simulink model "version5"  (R2018b)
settings: Solver=FixedStepAuto  StartTime=0.0  StopTime=1  FixedStep=0.0005  RelTol=1e-3  EnableMultiTasking=on
model workspace (MAT data in the model file):
  APPS_1_X = [526 863 1200 1537 1837 2212 2310]
  APPS_2_X = [0 342 684 1026 1368 1710 1805]
  APPS_Y = [100 80 60 40 20 0 0]
  Motor_Temp = [0 25 50 75 85 100 115 125 150 175 200 225 ... (13 elements, 1x13)]
  duty_time = [0 1000 5000 6500 7500 9000 10000 10000 10000 10000 10000 10000 ... (13 elements, 1x13)]
undefined symbols (not defined in the file): I_AN06_5V, I_AN08_5V, I_AN09_5V, I_HALL1, I_SW11_H, O_PWM1_LS0A7, O_PWM2_LS0A7, O_SW01_LS0A4
libraries: ec5744lib x55, simulink x28, canmsglib x12, fuzblock x2
(part 2 of 3)

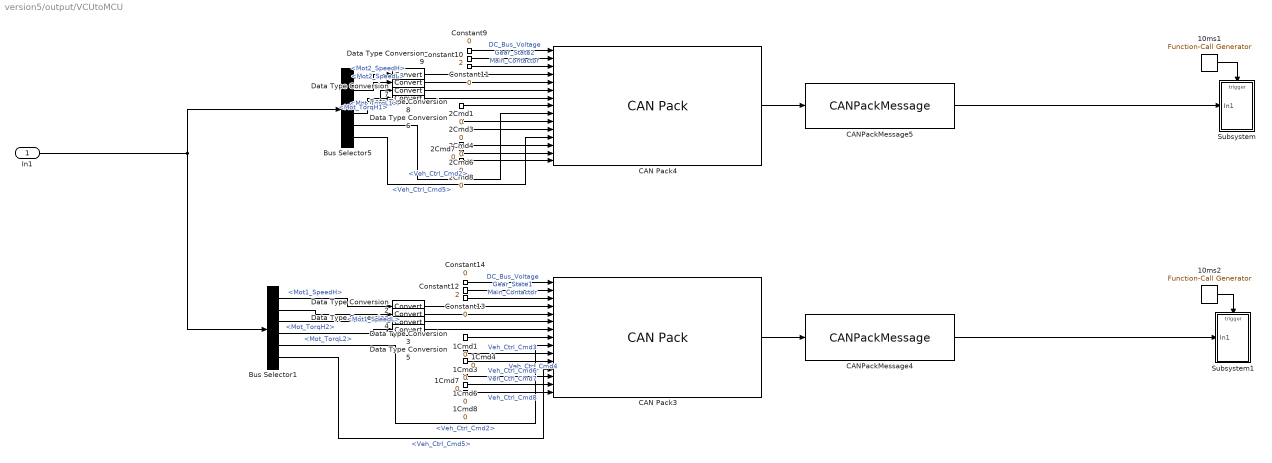
== system version5/output/VCUtoMCU ==
  In1 : Inport
  10ms1 : simulink/Ports & Subsystems/Function-Call Generator  sample_time=0.01  numberOfIterations=1
  10ms2 : simulink/Ports & Subsystems/Function-Call Generator  sample_time=0.01  numberOfIterations=1
  1Cmd{1,3..4,6..8} (6 alike) : Constant  Value=0
  2Cmd{1,3..4,6..8} (6 alike) : Constant  Value=0
  Bus Selector1 : BusSelector  OutputSignals=Mot1_SpeedH,Mot1_SpeedL,Mot_TorqH2,Mot_TorqL2,Veh_Ctrl_Cmd2,Veh_Ctrl_Cmd5
  Bus Selector5 : BusSelector  OutputSignals=Mot2_SpeedH,Mot2_SpeedL,Mot_TorqH1,Mot_TorqL1,Veh_Ctrl_Cmd2,Veh_Ctrl_Cmd5
  CAN Pack3 : canmsglib/CAN Pack  CANdbFile=C:\WH\MC.dbc  MsgList=VCUtoMCU1  MsgName=VCUtoMCU1  MsgIDType=Extended (29-bit identifier)  MsgIdentifier=146927393  MsgLength=8  SignalInfo=DC_Bus_Voltage$48$8$1$2$1$0$1$0$0$255$#Gear_State1$40$2$1$2$1$0$1$0$0$3$#Main_Montactor$43$1$1$2$1$0$1$0$0$1$#Mot1_Sp_H$0$8$1$2$1$0$5.000000e-01$-10000$-10000$-9.872500e+03$#Mot1_Sp_L$8$8$1$2$1$0$1$0$0$255$#Mot1_Torque_H$16$8$1$2$1$0$1$0$0$255$#Mot1_Torque_L$24$8$1$2$1$0$1$0$0$255$#Veh_Ctrl_Cmd1$32$1$1$2$1$0$1$0$0$1$#Veh_Ctrl_Cmd2$33$1$1$2$1$0$1$0$0$1$#Veh_Ctrl_Cmd3$34$1$1$2$1$0$1$0$0$1$#Veh_Ctrl_Cmd4$35$1$1$2$1$0$1$0$0$1$#Veh_Ctrl_Cmd5$36$1$1$2$1$0$1$0$0$1$#Veh_Ctrl_Cmd6$37$1$1$2$1$0$1$0$0$1$#Veh_Ctrl_Cmd7$38$1$1$2$1$0$1$0$0$1$#Veh_Ctrl_Cmd8$39$1$1$2$1$0$1$0$0$1$#  NSignals=15  StartBits=str2num('[int32(48);int32(40);int32(43);int32(0);int32(8);int32(16);int32(24);int32(32);int32(33);int32(34);int32(35);int32(36);int32(37);int32(38);int32(39)]')  SignalSizes=str2num('[int32(8);int32(2);int32(1);int32(8);int32(8);int32(8);int32(8);int32(1);int32(1);int32(1);int32(1);int32(1);int32(1);int32(1);int32(1)]')  ByteOrders=str2num('[int32(1);int32(1);int32(1);int32(1);int32(1);int32(1);int32(1);int32(1);int32(1);int32(1);int32(1);int32(1);int32(1);int32(1);int32(1)]')  DataTypes=str2num('[int32(2);int32(2);int32(2);int32(2);int32(2);int32(2);int32(2);int32(2);int32(2);int32(2);int32(2);int32(2);int32(2);int32(2);int32(2)]')  MultiplexTypes=str2num('[int32(1);int32(1);int32(1);int32(1);int32(1);int32(1);int32(1);int32(1);int32(1);int32(1);int32(1);int32(1);int32(1);int32(1);int32(1)]')  MultiplexValues=str2num('[double(0);double(0);double(0);double(0);double(0);double(0);double(0);double(0);double(0);double(0);double(0);double(0);double(0);double(0);double(0)]')  Factors=str2num('[double(1);double(1);double(1);double(5.000000e-01);double(1);double(1);double(1);double(1);double(1);double(1);double(1);double(1);double(1);double(1);double(1)]')  Offsets=str2num('[double(0);double(0);double(0);double(-10000);double(0);double(0);double(0);double(0);double(0);double(0);double(0);double(0);double(0);double(0);double(0)]')  Minimums=str2num('[double(0);double(0);double(0);double(-10000);double(0);double(0);double(0);double(0);double(0);double(0);double(0);double(0);double(0);double(0);double(0)]')  Maximums=str2num('[double(255);double(3);double(1);double(-9.872500e+03);double(255);double(255);double(255);double(1);double(1);double(1);double(1);double(1);double(1);double(1);double(1)]')  Remote=off  ApplyMinMax=off  BusOutput=off
      settings: SourceProductName=Simulink Real-Time  SourceProductBaseCode=XP  DataFormat=CANdb specified signals
  CAN Pack4 : canmsglib/CAN Pack  CANdbFile=C:\WH\MC.dbc  MsgList=VCUtoMCU2  MsgName=VCUtoMCU2  MsgIDType=Extended (29-bit identifier)  MsgIdentifier=145878817  MsgLength=8  SignalInfo=DC_Bus_Voltage$48$8$1$2$1$0$1$0$0$255$#Gear_State_2$40$2$1$2$1$0$1$0$0$3$#Main_Montactor$43$1$1$2$1$0$1$0$0$1$#Mot2_Sp_H$16$8$1$2$1$0$5.000000e-01$-10000$-10000$-9.872500e+03$#Mot2_Sp_L$24$8$1$2$1$0$5.000000e-01$-10000$-10000$-9.872500e+03$#Mot2_Torque_H$0$8$1$2$1$0$1$0$0$255$#Mot2_Torque_L$8$8$1$2$1$0$1$0$0$255$#Veh_Ctrl_Cmd1$32$1$1$2$1$0$1$0$0$1$#Veh_Ctrl_Cmd2$33$1$1$2$1$0$1$0$0$1$#Veh_Ctrl_Cmd3$34$1$1$2$1$0$1$0$0$1$#Veh_Ctrl_Cmd4$35$1$1$2$1$0$1$0$0$1$#Veh_Ctrl_Cmd5$36$1$1$2$1$0$1$0$0$1$#Veh_Ctrl_Cmd6$37$1$1$2$1$0$1$0$0$1$#Veh_Ctrl_Cmd7$38$1$1$2$1$0$1$0$0$1$#Veh_Ctrl_Cmd8$39$1$1$2$1$0$1$0$0$1$#  NSignals=15  StartBits=str2num('[int32(48);int32(40);int32(43);int32(16);int32(24);int32(0);int32(8);int32(32);int32(33);int32(34);int32(35);int32(36);int32(37);int32(38);int32(39)]')  SignalSizes=str2num('[int32(8);int32(2);int32(1);int32(8);int32(8);int32(8);int32(8);int32(1);int32(1);int32(1);int32(1);int32(1);int32(1);int32(1);int32(1)]')  ByteOrders=str2num('[int32(1);int32(1);int32(1);int32(1);int32(1);int32(1);int32(1);int32(1);int32(1);int32(1);int32(1);int32(1);int32(1);int32(1);int32(1)]')  DataTypes=str2num('[int32(2);int32(2);int32(2);int32(2);int32(2);int32(2);int32(2);int32(2);int32(2);int32(2);int32(2);int32(2);int32(2);int32(2);int32(2)]')  MultiplexTypes=str2num('[int32(1);int32(1);int32(1);int32(1);int32(1);int32(1);int32(1);int32(1);int32(1);int32(1);int32(1);int32(1);int32(1);int32(1);int32(1)]')  MultiplexValues=str2num('[double(0);double(0);double(0);double(0);double(0);double(0);double(0);double(0);double(0);double(0);double(0);double(0);double(0);double(0);double(0)]')  Factors=str2num('[double(1);double(1);double(1);double(5.000000e-01);double(5.000000e-01);double(1);double(1);double(1);double(1);double(1);double(1);double(1);double(1);double(1);double(1)]')  Offsets=str2num('[double(0);double(0);double(0);double(-10000);double(-10000);double(0);double(0);double(0);double(0);double(0);double(0);double(0);double(0);double(0);double(0)]')  Minimums=str2num('[double(0);double(0);double(0);double(-10000);double(-10000);double(0);double(0);double(0);double(0);double(0);double(0);double(0);double(0);double(0);double(0)]')  Maximums=str2num('[double(255);double(3);double(1);double(-9.872500e+03);double(-9.872500e+03);double(255);double(255);double(1);double(1);double(1);double(1);double(1);double(1);double(1);double(1)]')  Remote=off  ApplyMinMax=off  BusOutput=off
      settings: SourceProductName=Simulink Real-Time  SourceProductBaseCode=XP  DataFormat=CANdb specified signals
  CANPackMessage4 : ec5744lib/RapidECU_U3/04CANCommunication/CANPackMessage  datalength=8  sampletime=-1
      settings: SourceProductName=ECUCoder for MPC5744
  CANPackMessage5 : ec5744lib/RapidECU_U3/04CANCommunication/CANPackMessage  datalength=8  sampletime=-1
      settings: SourceProductName=ECUCoder for MPC5744
  Constant10 : Constant  Value=2
  Constant11 : Constant  Value=0
  Constant12 : Constant  Value=2  LockScale=on
  Constant13 : Constant  Value=0
  Constant14 : Constant  Value=0
  Constant9 : Constant  Value=0  OutDataTypeStr=uint8
  Data Type Conversion{2..9} (8 alike) : DataTypeConversion
  Subsystem : Subsystem
  Subsystem1 : Subsystem
  wires:
  Constant13/1 -> CAN Pack3/3  "Main_Contactor"
  1Cmd7/1 -> CAN Pack3/14  "Veh_Ctrl_Cmd7"
  CAN Pack3/1 -> CANPackMessage4/1
  Data Type Conversion2/1 -> CAN Pack3/4
  CAN Pack4/1 -> CANPackMessage5/1
  2Cmd7/1 -> CAN Pack4/14
  Constant10/1 -> CAN Pack4/2  "Gear_State2"
  1Cmd8/1 -> CAN Pack3/15  "Veh_Ctrl_Cmd8"
  2Cmd8/1 -> CAN Pack4/15
  Data Type Conversion5/1 -> CAN Pack3/7
  Constant12/1 -> CAN Pack3/2  "Gear_State1"
  CANPackMessage5/1 -> Subsystem/1(In1)
  2Cmd6/1 -> CAN Pack4/13
  1Cmd4/1 -> CAN Pack3/11  "Veh_Ctrl_Cmd4"
  Data Type Conversion7/1 -> CAN Pack4/6
  Constant14/1 -> CAN Pack3/1  "DC_Bus_Voltage"
  Data Type Conversion3/1 -> CAN Pack3/5
  1Cmd3/1 -> CAN Pack3/10  "Veh_Ctrl_Cmd3"
  Constant9/1 -> CAN Pack4/1  "DC_Bus_Voltage"
  Bus Selector5/5 -> CAN Pack4/9  "<Veh_Ctrl_Cmd2>"
  1Cmd6/1 -> CAN Pack3/13  "Veh_Ctrl_Cmd6"
  10ms2/1 -> Subsystem1/Trigger
  Constant11/1 -> CAN Pack4/3  "Main_Contactor"
  2Cmd4/1 -> CAN Pack4/11
  Bus Selector5/6 -> CAN Pack4/12  "<Veh_Ctrl_Cmd5>"
  In1/1 -> Bus Selector5/1, Bus Selector1/1
  2Cmd1/1 -> CAN Pack4/8
  Bus Selector5/1 -> Data Type Conversion9/1  "<Mot2_SpeedH>"
  CANPackMessage4/1 -> Subsystem1/1(In1)
  Bus Selector1/5 -> CAN Pack3/9  "<Veh_Ctrl_Cmd2>"
  2Cmd3/1 -> CAN Pack4/10
  Data Type Conversion4/1 -> CAN Pack3/6
  10ms1/1 -> Subsystem/Trigger
  Data Type Conversion8/1 -> CAN Pack4/5
  Bus Selector1/3 -> Data Type Conversion4/1  "<Mot_TorqH2>"
  Bus Selector1/4 -> Data Type Conversion5/1  "<Mot_TorqL2>"
  Bus Selector5/4 -> Data Type Conversion6/1  "<Mot_TorqL1>"
  Data Type Conversion9/1 -> CAN Pack4/4
  1Cmd1/1 -> CAN Pack3/8
  Bus Selector1/1 -> Data Type Conversion2/1  "<Mot1_SpeedH>"
  Bus Selector1/2 -> Data Type Conversion3/1  "<Mot1_SpeedL>"
  Bus Selector1/6 -> CAN Pack3/12  "<Veh_Ctrl_Cmd5>"
  Bus Selector5/2 -> Data Type Conversion8/1  "<Mot2_SpeedL>"
  Data Type Conversion6/1 -> CAN Pack4/7
  Bus Selector5/3 -> Data Type Conversion7/1  "<Mot_TorqH1>"

== system version5/control/APS_Ctrl/clock ==
  In1 : Inport
  AND : Logic  IconShape=distinctive  AllPortsSameDT=off  OutDataTypeStr=boolean
  Compare To Constant : simulink/Logic and Bit Operations/Compare To Constant  relop===  const=1  OutDataTypeStr=boolean
  Compare To Constant1 : simulink/Logic and Bit Operations/Compare To Constant  relop===  const=1  OutDataTypeStr=boolean
  计时计数 : Subsystem  Description=计数模块，当有输入信号有跳变的时候会触发使计数值清零  TreatAsAtomicUnit=on
  Out1 : Outport
  wires:
  Compare To Constant1/1 -> AND/2
  Compare To Constant/1 -> AND/1
  计时计数/1(Count_state) -> Compare To Constant/1
  In1/1 -> 计时计数/1(计数状态), Compare To Constant1/1
  AND/1 -> Out1/1

== system version5/control/tcs/0-75直线加速 ==
  In1 : Inport
  In2 : Inport  Port=2
  In3 : Inport  Port=3
  1-D Lookup Table : Lookup_n-D  NumberOfTableDimensions=1  BreakpointsForDimension1=[1 256 512 768 1024 1280 1536 1792 2048 2304 2560 2816 3072 3328 3584 3840 4096 4352 4608 4864 5120 5376 5632 5888 6000]  Table=[134 134 134 134 134 134 134 134 134 134 134 134 134 134 134 134 134 134 132 130 128 125 120 117 115]  InternalRulePriority=Speed  RndMeth=Simplest  InputSameDT=on
  1-D Lookup Table1 : Lookup_n-D  NumberOfTableDimensions=1  BreakpointsForDimension1=[1 256 512 768 1024 1280 1536 1792 2048 2304 2560 2816 3072 3328 3584 3840 4096 4352 4608 4864 5120 5376 5632 5888 6000]  Table=[134 134 134 134 134 134 134 134 134 134 134 134 134 134 134 134 134 134 132 130 128 125 120 117 115]  InternalRulePriority=Speed  RndMeth=Simplest  InputSameDT=on
  "ACC " : Fcn  Expr=u(1)^(0.7)
  Dot Product4 : DotProduct  InputSameDT=on  OutDataTypeStr=Inherit: Inherit via internal rule
  Gain2 : Gain  Gain=0.5  OutDataTypeStr=double
  Subtract1 : Sum  AccumDataTypeStr=double  OutDataTypeStr=uint16  SaturateOnIntegerOverflow=on
  Out1 : Outport
  Output : Outport  Port=2
  wires:
  Dot Product4/1 -> Out1/1
  In2/1 -> 1-D Lookup Table/1
  Subtract1/1 -> Gain2/1
  1-D Lookup Table1/1 -> Subtract1/2
  In3/1 -> 1-D Lookup Table1/1
  "ACC "/1 -> Dot Product4/2
  In1/1 -> "ACC "/1
  1-D Lookup Table/1 -> Subtract1/1
  Gain2/1 -> Output/1, Dot Product4/1

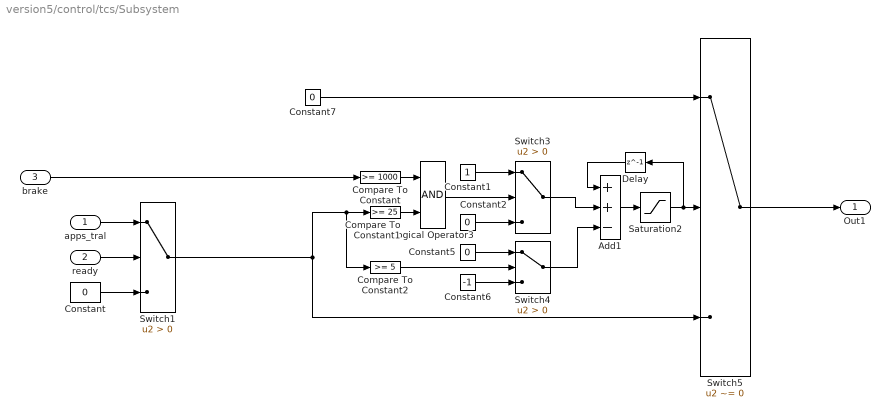
== system version5/control/tcs/Subsystem ==
  apps_tral : Inport
  ready : Inport  Port=2
  brake : Inport  Port=3
  Add1 : Sum  Inputs=++-
  Compare To Constant : simulink/Logic and Bit Operations/Compare To Constant  relop=>=  const=1000  OutDataTypeStr=boolean
  Compare To Constant1 : simulink/Logic and Bit Operations/Compare To Constant  relop=>=  const=25  OutDataTypeStr=boolean
  Compare To Constant2 : simulink/Logic and Bit Operations/Compare To Constant  relop=>=  const=5  OutDataTypeStr=boolean
  Constant{,2,5,7} (4 alike) : Constant  Value=0
  Constant1 : Constant
  Constant6 : Constant  Value=-1
  Delay : Delay  DelayLength=1  InitialCondition=0
  Logical Operator3 : Logic  AllPortsSameDT=off  OutDataTypeStr=boolean
  Saturation2 : Saturate  UpperLimit=1  LowerLimit=0  OutDataTypeStr=single
  Switch1 : Switch  Criteria=u2 > Threshold
  Switch3 : Switch  Criteria=u2 > Threshold  OutDataTypeStr=single
  Switch4 : Switch  Criteria=u2 > Threshold  OutDataTypeStr=single
  Switch5 : Switch  Criteria=u2 ~= 0  OutDataTypeStr=uint16
  Out1 : Outport
  wires:
  Switch4/1 -> Add1/3
  Constant/1 -> Switch1/3
  Switch1/1 -> Compare To Constant2/1, Compare To Constant1/1, Switch5/3
  Constant5/1 -> Switch4/1
  Constant2/1 -> Switch3/3
  apps_tral/1 -> Switch1/1
  Constant6/1 -> Switch4/3
  Delay/1 -> Add1/1
  Compare To Constant1/1 -> Logical Operator3/2
  Add1/1 -> Saturation2/1
  Compare To Constant2/1 -> Switch4/2
  Switch3/1 -> Add1/2
  Compare To Constant/1 -> Logical Operator3/1
  Constant7/1 -> Switch5/1
  Saturation2/1 -> Delay/1, Switch5/2
  Logical Operator3/1 -> Switch3/2
  Constant1/1 -> Switch3/1
  brake/1 -> Compare To Constant/1
  Switch5/1 -> Out1/1
  ready/1 -> Switch1/2

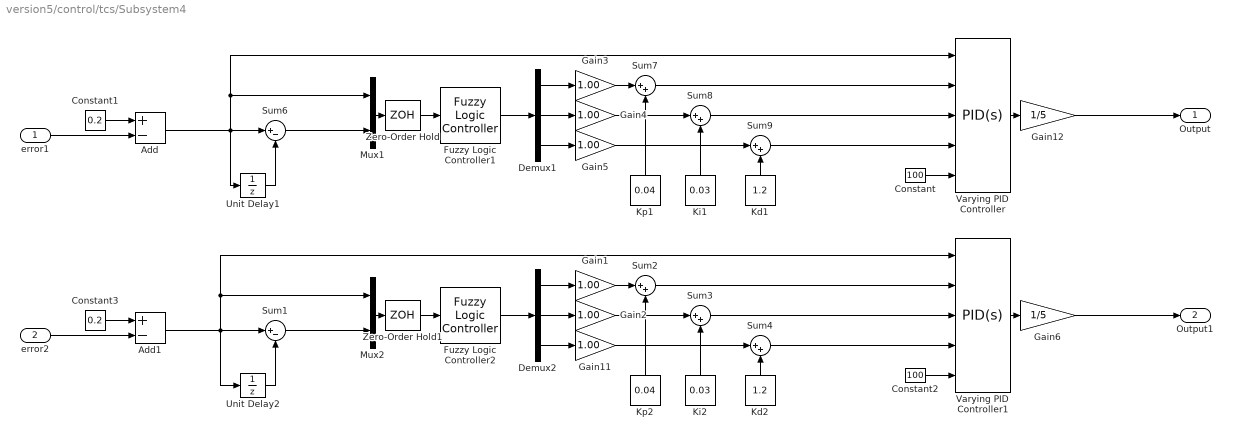
== system version5/control/tcs/Subsystem4 ==
  error1 : Inport
  error2 : Inport  Port=2
  Add : Sum  Inputs=+-
  Add1 : Sum  Inputs=+-
  Constant : Constant  Value=100
  Constant1 : Constant  Value=0.2
  Constant2 : Constant  Value=100
  Constant3 : Constant  Value=0.2
  Demux1 : Demux  Outputs=3
  Demux2 : Demux  Outputs=3
  Fuzzy Logic Controller1 : fuzblock/Fuzzy Logic  Controller  FIS='myfuzzyrules.fis'  OutputSampleNumber=101  DataType=double  FuzzifiedInputs=off  RuleFiringStrengths=off  RuleOutputs=off  AggregatedOutputs=off  SimulateUsing=Interpreted execution  OutOfRangeInputValueMessage=warning  NoRuleFiredMessage=warning  EmptyOutputFuzzySetMessage=warning
  Fuzzy Logic Controller2 : fuzblock/Fuzzy Logic  Controller  FIS='myfuzzyrules.fis'  OutputSampleNumber=101  DataType=double  FuzzifiedInputs=off  RuleFiringStrengths=off  RuleOutputs=off  AggregatedOutputs=off  SimulateUsing=Interpreted execution  OutOfRangeInputValueMessage=warning  NoRuleFiredMessage=warning  EmptyOutputFuzzySetMessage=warning
  Gain{1..5,11} (6 alike) : Gain  Gain=1.00
  Gain12 : Gain  Gain=1/5
  Gain6 : Gain  Gain=1/5
  Kd1 : Constant  Value=1.2
  Kd2 : Constant  Value=1.2
  Ki1 : Constant  Value=0.03
  Ki2 : Constant  Value=0.03
  Kp1 : Constant  Value=0.04
  Kp2 : Constant  Value=0.04
  Mux1 : Mux  Inputs=2
  Mux2 : Mux  Inputs=2
  Sum1 : Sum  Inputs=|+-
  Sum{2..4,7..9} (6 alike) : Sum  Inputs=|++
  Sum6 : Sum  Inputs=|+-
  Unit Delay1 : UnitDelay  SampleTime=-1
  Unit Delay2 : UnitDelay  SampleTime=-1
  Varying PID Controller : simulink/Continuous/PID Controller  Controller=PID  Form=Parallel  TimeDomain=Continuous-time  SampleTime=-1  IntegratorMethod=Forward Euler  FilterMethod=Forward Euler  ControllerParametersSource=external  P=1  I=1  D=0  UseFilter=on  N=100  TunerSelectOption=Transfer Function Based (PID Tuner App)  InitialConditionSource=internal  InitialConditionForIntegrator=0  InitialConditionForFilter=0  DifferentiatorICPrevScaledInput=0  ExternalReset=none  TrackingMode=off  Kt=1  LimitOutput=off  UpperSaturationLimit=inf  LowerSaturationLimit=-inf  LinearizeAsGain=on  AntiWindupMode=none  Kb=1  POutMin=[]  POutMax=[]  IOutMin=[]  IOutMax=[]  DOutMin=[]  DOutMax=[]  NOutMin=[]  NOutMax=[]  SumOutMin=[]  SumOutMax=[]  SaturationOutMin=[]  SaturationOutMax=[]  PParamMin=[]  PParamMax=[]  IParamMin=[]  IParamMax=[]  DParamMin=[]  DParamMax=[]  NParamMin=[]  NParamMax=[]  KbParamMin=[]  KbParamMax=[]  KtParamMin=[]  KtParamMax=[]  KbOutMin=[]  KbOutMax=[]  KtOutMin=[]  KtOutMax=[]  IntegratorOutMin=[]  IntegratorOutMax=[]  FilterOutMin=[]  FilterOutMax=[]  SumI1OutMin=[]  SumI1OutMax=[]  SumI2OutMin=[]  SumI2OutMax=[]  SumI3OutMin=[]  SumI3OutMax=[]  SumI4OutMin=[]  SumI4OutMax=[]  SumDOutMin=[]  SumDOutMax=[]  DifferentiatorOutMin=[]  DifferentiatorOutMax=[]  FilterDiffOutCoefMin=[]  FilterDiffOutCoefMax=[]  ReciprocalOutMin=[]  ReciprocalOutMax=[]  SumDenOutMin=[]  SumDenOutMax=[]  SumNumOutMin=[]  SumNumOutMax=[]  DivideOutMin=[]  DivideOutMax=[]  IntegratorContinuousStateAttributes=''  IntegratorStateMustResolveToSignalObject=off  IntegratorRTWStateStorageClass=Auto  FilterContinuousStateAttributes=''  FilterStateMustResolveToSignalObject=off  FilterRTWStateStorageClass=Auto  ParallelPVariant=ExternalParameters  IdealPVariant=Disabled  IVariant=ExternalParameters  DVariant=ExternalParameters  IntegratorVariant=Continuous  SatVariant=Disabled  AWVariant=Passthrough  PCopyVariant=Disabled  TRVariant=Disabled  FdbkBlocksVariant=Forward  IdealPFdbkVariant=Disabled  SatFdbkVariant=Disabled  DerivativeFilterVariant=ContFilter  NVariant=ExternalParameters  NCopyVariant=Disabled  FilterICVariant=InternalICsFilter  IntegratorICVariant=InternalICs  ExternalResetVariant=Disabled  TRSumVariant=Passthrough  SumFdbkVariant=Disabled  SumVariant=Sum_PID
  Varying PID Controller1 : simulink/Continuous/PID Controller  Controller=PID  Form=Parallel  TimeDomain=Continuous-time  SampleTime=-1  IntegratorMethod=Forward Euler  FilterMethod=Forward Euler  ControllerParametersSource=external  P=1  I=1  D=0  UseFilter=on  N=100  TunerSelectOption=Transfer Function Based (PID Tuner App)  InitialConditionSource=internal  InitialConditionForIntegrator=0  InitialConditionForFilter=0  DifferentiatorICPrevScaledInput=0  ExternalReset=none  TrackingMode=off  Kt=1  LimitOutput=off  UpperSaturationLimit=inf  LowerSaturationLimit=-inf  LinearizeAsGain=on  AntiWindupMode=none  Kb=1  POutMin=[]  POutMax=[]  IOutMin=[]  IOutMax=[]  DOutMin=[]  DOutMax=[]  NOutMin=[]  NOutMax=[]  SumOutMin=[]  SumOutMax=[]  SaturationOutMin=[]  SaturationOutMax=[]  PParamMin=[]  PParamMax=[]  IParamMin=[]  IParamMax=[]  DParamMin=[]  DParamMax=[]  NParamMin=[]  NParamMax=[]  KbParamMin=[]  KbParamMax=[]  KtParamMin=[]  KtParamMax=[]  KbOutMin=[]  KbOutMax=[]  KtOutMin=[]  KtOutMax=[]  IntegratorOutMin=[]  IntegratorOutMax=[]  FilterOutMin=[]  FilterOutMax=[]  SumI1OutMin=[]  SumI1OutMax=[]  SumI2OutMin=[]  SumI2OutMax=[]  SumI3OutMin=[]  SumI3OutMax=[]  SumI4OutMin=[]  SumI4OutMax=[]  SumDOutMin=[]  SumDOutMax=[]  DifferentiatorOutMin=[]  DifferentiatorOutMax=[]  FilterDiffOutCoefMin=[]  FilterDiffOutCoefMax=[]  ReciprocalOutMin=[]  ReciprocalOutMax=[]  SumDenOutMin=[]  SumDenOutMax=[]  SumNumOutMin=[]  SumNumOutMax=[]  DivideOutMin=[]  DivideOutMax=[]  IntegratorContinuousStateAttributes=''  IntegratorStateMustResolveToSignalObject=off  IntegratorRTWStateStorageClass=Auto  FilterContinuousStateAttributes=''  FilterStateMustResolveToSignalObject=off  FilterRTWStateStorageClass=Auto  ParallelPVariant=ExternalParameters  IdealPVariant=Disabled  IVariant=ExternalParameters  DVariant=ExternalParameters  IntegratorVariant=Continuous  SatVariant=Disabled  AWVariant=Passthrough  PCopyVariant=Disabled  TRVariant=Disabled  FdbkBlocksVariant=Forward  IdealPFdbkVariant=Disabled  SatFdbkVariant=Disabled  DerivativeFilterVariant=ContFilter  NVariant=ExternalParameters  NCopyVariant=Disabled  FilterICVariant=InternalICsFilter  IntegratorICVariant=InternalICs  ExternalResetVariant=Disabled  TRSumVariant=Passthrough  SumFdbkVariant=Disabled  SumVariant=Sum_PID
  Zero-Order Hold : ZeroOrderHold  SampleTime=-1
  Zero-Order Hold1 : ZeroOrderHold  SampleTime=-1
  Output : Outport
  Output1 : Outport  Port=2
  wires:
  Sum9/1 -> Varying PID Controller/4
  Gain4/1 -> Sum8/1
  Sum8/1 -> Varying PID Controller/3
  Constant1/1 -> Add/1
  Gain3/1 -> Sum7/1
  Fuzzy Logic Controller1/1 -> Demux1/1
  Demux1/1 -> Gain3/1
  Unit Delay1/1 -> Sum6/2
  Kd1/1 -> Sum9/2
  Demux1/2 -> Gain4/1
  Kp1/1 -> Sum7/2
  Sum7/1 -> Varying PID Controller/2
  Gain5/1 -> Sum9/1
  error1/1 -> Add/2
  Demux1/3 -> Gain5/1
  Ki1/1 -> Sum8/2
  Constant/1 -> Varying PID Controller/5
  Sum2/1 -> Varying PID Controller1/2
  Sum3/1 -> Varying PID Controller1/3
  Sum4/1 -> Varying PID Controller1/4
  Constant3/1 -> Add1/1
  Demux2/2 -> Gain2/1
  Demux2/3 -> Gain11/1
  Unit Delay2/1 -> Sum1/2
  Gain11/1 -> Sum4/1
  Kp2/1 -> Sum2/2
  Demux2/1 -> Gain1/1
  Gain1/1 -> Sum2/1
  Fuzzy Logic Controller2/1 -> Demux2/1
  Ki2/1 -> Sum3/2
  Kd2/1 -> Sum4/2
  Constant2/1 -> Varying PID Controller1/5
  Gain2/1 -> Sum3/1
  Varying PID Controller1/1 -> Gain6/1
  error2/1 -> Add1/2
  Varying PID Controller/1 -> Gain12/1
  Gain12/1 -> Output/1
  Gain6/1 -> Output1/1
  Sum6/1 -> Mux1/2
  Sum1/1 -> Mux2/2
  Add/1 -> Varying PID Controller/1, Mux1/1, Unit Delay1/1, Sum6/1
  Add1/1 -> Mux2/1, Varying PID Controller1/1, Unit Delay2/1, Sum1/1
  Zero-Order Hold/1 -> Fuzzy Logic Controller1/1
  Mux1/1 -> Zero-Order Hold/1
  Zero-Order Hold1/1 -> Fuzzy Logic Controller2/1
  Mux2/1 -> Zero-Order Hold1/1

== system version5/control/tcs/均值滤波器 ==
  In1 : Inport
  Add2 : Sum  Inputs=-+-
  Constant2 : Constant  Value=4  OutDataTypeStr=uint8  SampleTime=-1
  Divide : Product  Inputs=*/
  MinMax : MinMax
  MinMax1 : MinMax  Function=max
  Sum of Elements : Sum  Inputs=+
  Tapped Delay : simulink/Discrete/Tapped Delay  vinit=0.0  samptime=-1  NumDelays=4  DelayOrder=Oldest  includeCurrent=off
  Out1 : Outport
  wires:
  In1/1 -> Tapped Delay/1
  Add2/1 -> Divide/1
  MinMax/1 -> Add2/3
  MinMax1/1 -> Add2/1
  Divide/1 -> Out1/1
  Constant2/1 -> Divide/2
  Sum of Elements/1 -> Add2/2
  Tapped Delay/1 -> MinMax/1, MinMax1/1, Sum of Elements/1

== system version5/control/tcs/均值滤波器1 ==
  In1 : Inport
  Add2 : Sum  Inputs=-+-
  Constant2 : Constant  Value=4  OutDataTypeStr=uint8  SampleTime=-1
  Divide : Product  Inputs=*/
  MinMax : MinMax
  MinMax1 : MinMax  Function=max
  Sum of Elements : Sum  Inputs=+
  Tapped Delay : simulink/Discrete/Tapped Delay  vinit=0.0  samptime=-1  NumDelays=4  DelayOrder=Oldest  includeCurrent=off
  Out1 : Outport
  wires:
  Tapped Delay/1 -> Sum of Elements/1, MinMax1/1, MinMax/1
  Sum of Elements/1 -> Add2/2
  Constant2/1 -> Divide/2
  Divide/1 -> Out1/1
  MinMax1/1 -> Add2/1
  MinMax/1 -> Add2/3
  Add2/1 -> Divide/1
  In1/1 -> Tapped Delay/1

== system version5/control/tcs/均值滤波器2 ==
  In1 : Inport
  Add2 : Sum  Inputs=-+-
  Constant2 : Constant  Value=4  OutDataTypeStr=uint8  SampleTime=-1
  Divide : Product  Inputs=*/
  MinMax : MinMax
  MinMax1 : MinMax  Function=max
  Sum of Elements : Sum  Inputs=+
  Tapped Delay : simulink/Discrete/Tapped Delay  vinit=0.0  samptime=-1  NumDelays=4  DelayOrder=Oldest  includeCurrent=off
  Out1 : Outport
  wires:
  In1/1 -> Tapped Delay/1
  Add2/1 -> Divide/1
  MinMax/1 -> Add2/3
  MinMax1/1 -> Add2/1
  Divide/1 -> Out1/1
  Constant2/1 -> Divide/2
  Sum of Elements/1 -> Add2/2
  Tapped Delay/1 -> MinMax/1, MinMax1/1, Sum of Elements/1

== system version5/control/tcs/持续模式 ==
  In1 : Inport
  In2 : Inport  Port=2
  In3 : Inport  Port=3
  1-D Lookup Table : Lookup_n-D  NumberOfTableDimensions=1  BreakpointsForDimension1=[0 300 600 900 1200 1500 1800 2100 2400 2700 3000 3300 3600 3900 4200 4500 4800 5100 5400 5700 6000]  Table=[60 60 61 62 62 63 63 64 65 64 63 62 62 61 61 60 59 58 57 56 55]  InternalRulePriority=Speed  RndMeth=Simplest  InputSameDT=on
  1-D Lookup Table1 : Lookup_n-D  NumberOfTableDimensions=1  BreakpointsForDimension1=[0 300 600 900 1200 1500 1800 2100 2400 2700 3000 3300 3600 3900 4200 4500 4800 5100 5400 5700 6000]  Table=[60 60 61 62 62 63 63 64 65 64 63 62 62 61 61 60 59 58 57 56 55]  InternalRulePriority=Speed  RndMeth=Simplest  InputSameDT=on
  ACC : Fcn  Expr=u(1)
  Dot Product5 : DotProduct  InputSameDT=on  OutDataTypeStr=Inherit: Inherit via internal rule
  Gain3 : Gain  Gain=0.5  OutDataTypeStr=double
  Subtract2 : Sum  AccumDataTypeStr=double  OutDataTypeStr=uint16  SaturateOnIntegerOverflow=on
  Out1 : Outport
  wires:
  In2/1 -> 1-D Lookup Table/1
  1-D Lookup Table1/1 -> Subtract2/2
  Gain3/1 -> Dot Product5/2
  1-D Lookup Table/1 -> Subtract2/1
  In3/1 -> 1-D Lookup Table1/1
  In1/1 -> ACC/1
  Subtract2/1 -> Gain3/1
  Dot Product5/1 -> Out1/1
  ACC/1 -> Dot Product5/1

== system version5/input/AnalogInput/Acc Pedal Gather ==
  function : TriggerPort  TriggerType=function-call  VariantControl=Variant
  AnalogInput1 : ec5744lib/RapidECU_U3/01BasicInput/AnalogInput  channel=55:I_AN09_5V  sampletime=-1
      settings: SourceProductName=ECUCoder for MPC5744
  AnalogInput2 : ec5744lib/RapidECU_U3/01BasicInput/AnalogInput  channel=54:I_AN08_5V  sampletime=-1
      settings: SourceProductName=ECUCoder for MPC5744
  APPS_1 : Outport
  APPS_2 : Outport  Port=2
  wires:
  AnalogInput2/1 -> APPS_1/1  "APPS_1"
  AnalogInput1/1 -> APPS_2/1  "APPS_2"

== system version5/input/AnalogInput/Brake Pedal Gather ==
  function : TriggerPort  TriggerType=function-call  VariantControl=Variant
  AnalogInput : ec5744lib/RapidECU_U3/01BasicInput/AnalogInput  channel=52:I_AN06_5V  sampletime=-1
      settings: SourceProductName=ECUCoder for MPC5744
  Brake : Outport
  wires:
  AnalogInput/1 -> Brake/1  "Brake"

== system version5/input/BMStoVCU/Function-Call Subsystem ==
  CAN_OK : Inport
  ID : Inport  Port=2
  Msg : Inport  Port=3
  function : TriggerPort  TriggerType=function-call  VariantControl=Variant
  Enabled Subsystem : Subsystem  TreatAsAtomicUnit=on
  Bat_Ala_Lv : Outport
  Bat_Current_LSB : Outport  Port=2
  Bat_Current_MSB : Outport  Port=3
  Bat_Stat : Outport  Port=4
  Bat_Voltage_LSB : Outport  Port=5
  Bat_Valtage_MSB : Outport  Port=6
  Bat_soc : Outport  Port=7
  wires:
  CAN_OK/1 -> Enabled Subsystem/Enable
  ID/1 -> Enabled Subsystem/1(ID)
  Msg/1 -> Enabled Subsystem/2(Msg)
  Enabled Subsystem/1(Bat_Ala_Lv) -> Bat_Ala_Lv/1
  Enabled Subsystem/7(Bat_soc) -> Bat_soc/1
  Enabled Subsystem/6(Bat_Valtage_MSB) -> Bat_Valtage_MSB/1
  Enabled Subsystem/5(Bat_Voltage_LSB) -> Bat_Voltage_LSB/1
  Enabled Subsystem/4(Bat_Stat) -> Bat_Stat/1
  Enabled Subsystem/3(Bat_Current_MSB) -> Bat_Current_MSB/1
  Enabled Subsystem/2(Bat_Current_LSB) -> Bat_Current_LSB/1

== system version5/input/BMStoVCU/Function-Call Subsystem1 ==
  CAN_OK : Inport
  ID : Inport  Port=2
  Msg : Inport  Port=3
  function : TriggerPort  TriggerType=function-call  VariantControl=Variant
  Enabled Subsystem : Subsystem  TreatAsAtomicUnit=on
  Bat_Max_Temp : Outport
  wires:
  CAN_OK/1 -> Enabled Subsystem/Enable
  ID/1 -> Enabled Subsystem/1(ID)
  Msg/1 -> Enabled Subsystem/2(Msg)
  Enabled Subsystem/1(Bat_Max_Temp) -> Bat_Max_Temp/1

== system version5/input/DASHtoVCU/Function-Call Subsystem6 ==
  CAN_OK : Inport
  ID : Inport  Port=2
  Msg : Inport  Port=3
  function : TriggerPort  TriggerType=function-call  VariantControl=Variant
  Enabled Subsystem : Subsystem  TreatAsAtomicUnit=on
  GEAR : Outport
  Key_For_Dash : Outport  Port=2
  wires:
  Enabled Subsystem/2(Key_For_Dash) -> Key_For_Dash/1
  Enabled Subsystem/1(GEAR) -> GEAR/1
  Msg/1 -> Enabled Subsystem/2(Msg)
  ID/1 -> Enabled Subsystem/1(ID)
  CAN_OK/1 -> Enabled Subsystem/Enable

== system version5/input/MCU to VCU/Function-Call Subsystem2 ==
  CAN_OK : Inport
  ID : Inport  Port=2
  Msg : Inport  Port=3
  function : TriggerPort  TriggerType=function-call  VariantControl=Variant
  Enabled Subsystem : Subsystem  TreatAsAtomicUnit=on
  Mot1_Sp_H : Outport
  Mot1_Sp_L : Outport  Port=2
  Mot1_Torque_H : Outport  Port=3
  Mot1_Torque_L : Outport  Port=4
  Veh_Ctrl_Cmd2 : Outport  Port=5
  Veh_Ctrl_Cmd5 : Outport  Port=6
  wires:
  CAN_OK/1 -> Enabled Subsystem/Enable
  ID/1 -> Enabled Subsystem/1(ID)
  Msg/1 -> Enabled Subsystem/2(Msg)
  Enabled Subsystem/4(Mot1_Torque_L) -> Mot1_Torque_L/1
  Enabled Subsystem/3(Mot1_Torque_H) -> Mot1_Torque_H/1
  Enabled Subsystem/2(Mot1_Sp_L) -> Mot1_Sp_L/1
  Enabled Subsystem/1(Mot1_Sp_H) -> Mot1_Sp_H/1
  Enabled Subsystem/6(Veh_Ctrl_Cmd5) -> Veh_Ctrl_Cmd5/1
  Enabled Subsystem/5(Veh_Ctrl_Cmd2) -> Veh_Ctrl_Cmd2/1

== system version5/input/MCU to VCU/Function-Call Subsystem3 ==
  CAN_OK : Inport
  ID : Inport  Port=2
  Msg : Inport  Port=3
  function : TriggerPort  TriggerType=function-call  VariantControl=Variant
  Enabled Subsystem : Subsystem  TreatAsAtomicUnit=on
  Mot2_Sp_H : Outport
  Mot2_Sp_L : Outport  Port=2
  Mot2_Torque_H : Outport  Port=3
  Mot2_Torque_L : Outport  Port=4
  Veh_Ctrl_Cmd2 : Outport  Port=5
  Veh_Ctrl_Cmd5 : Outport  Port=6
  wires:
  CAN_OK/1 -> Enabled Subsystem/Enable
  ID/1 -> Enabled Subsystem/1(ID)
  Msg/1 -> Enabled Subsystem/2(Msg)
  Enabled Subsystem/1(Mot2_Sp_H) -> Mot2_Sp_H/1
  Enabled Subsystem/2(Mot2_Sp_L) -> Mot2_Sp_L/1
  Enabled Subsystem/3(Mot2_Torque_H) -> Mot2_Torque_H/1
  Enabled Subsystem/4(Mot2_Torque_L) -> Mot2_Torque_L/1
  Enabled Subsystem/5(Veh_Ctrl_Cmd2) -> Veh_Ctrl_Cmd2/1
  Enabled Subsystem/6(Veh_Ctrl_Cmd5) -> Veh_Ctrl_Cmd5/1

== system version5/input/MCUtoVCU/Function-Call Subsystem4 ==
  CAN_OK : Inport
  ID : Inport  Port=2
  Msg : Inport  Port=3
  function : TriggerPort  TriggerType=function-call  VariantControl=Variant
  Enabled Subsystem : Subsystem  TreatAsAtomicUnit=on
  MCU_Temp1 : Outport
  Motor_Temp1 : Outport  Port=2
  wires:
  CAN_OK/1 -> Enabled Subsystem/Enable
  ID/1 -> Enabled Subsystem/1(ID)
  Msg/1 -> Enabled Subsystem/2(Msg)
  Enabled Subsystem/1(MCU_Temp1) -> MCU_Temp1/1
  Enabled Subsystem/2(Motor_Temp1) -> Motor_Temp1/1

== system version5/input/MCUtoVCU/Function-Call Subsystem5 ==
  CAN_OK : Inport
  ID : Inport  Port=2
  Msg : Inport  Port=3
  function : TriggerPort  TriggerType=function-call  VariantControl=Variant
  Enabled Subsystem : Subsystem  TreatAsAtomicUnit=on
  MCU_Temp2 : Outport
  Motor_Temp2 : Outport  Port=2
  wires:
  CAN_OK/1 -> Enabled Subsystem/Enable
  ID/1 -> Enabled Subsystem/1(ID)
  Msg/1 -> Enabled Subsystem/2(Msg)
  Enabled Subsystem/1(MCU_Temp2) -> MCU_Temp2/1
  Enabled Subsystem/2(Motor_Temp2) -> Motor_Temp2/1

== system version5/output/Subsystem/Subsystem2 ==
  In1 : Inport
  function : TriggerPort  TriggerType=function-call  VariantControl=Variant
  CANTransmit5 : ec5744lib/RapidECU_U3/04CANCommunication/CANTransmit  canmodule=1  canbuffer=8  canmessageid=hex2dec('211')  canmessagetype=Standard(11-bit ID)  datalength=8  sampletime=-1
      settings: SourceProductName=ECUCoder for MPC5744
  MeaModule2 : ec5744lib/RapidECU_U3/07Calibration/MeaModule  signal=VCUtoDASH_Pow
      settings: SourceProductName=ECUCoder for MPC5744
  Terminator12 : Terminator
  wires:
  CANTransmit5/1 -> MeaModule2/1
  In1/1 -> CANTransmit5/1
  MeaModule2/1 -> Terminator12/1

== system version5/output/Subsystem/Subsystem3 ==
  In1 : Inport
  function : TriggerPort  TriggerType=function-call  VariantControl=Variant
  CANTransmit1 : ec5744lib/RapidECU_U3/04CANCommunication/CANTransmit  canmodule=2  canbuffer=9  canmessageid=hex2dec('213')  canmessagetype=Standard(11-bit ID)  datalength=8  sampletime=-1
      settings: SourceProductName=ECUCoder for MPC5744
  MeaModule3 : ec5744lib/RapidECU_U3/07Calibration/MeaModule  signal=VCUtoDASH_Bat
      settings: SourceProductName=ECUCoder for MPC5744
  Terminator : Terminator
  wires:
  CANTransmit1/1 -> MeaModule3/1
  MeaModule3/1 -> Terminator/1
  In1/1 -> CANTransmit1/1

== system version5/output/Subsystem/Subsystem4 ==
  In1 : Inport
  function : TriggerPort  TriggerType=function-call  VariantControl=Variant
  CANTransmit2 : ec5744lib/RapidECU_U3/04CANCommunication/CANTransmit  canmodule=2  canbuffer=8  canmessageid=hex2dec('212')  canmessagetype=Standard(11-bit ID)  datalength=8  sampletime=-1
      settings: SourceProductName=ECUCoder for MPC5744
  MeaModule4 : ec5744lib/RapidECU_U3/07Calibration/MeaModule  signal=VCUtoDASH_Mot
      settings: SourceProductName=ECUCoder for MPC5744
  Terminator1 : Terminator
  wires:
  In1/1 -> CANTransmit2/1
  MeaModule4/1 -> Terminator1/1
  CANTransmit2/1 -> MeaModule4/1

== system version5/output/VCUtoMCU/Subsystem ==
  In1 : Inport
  function : TriggerPort  TriggerType=function-call  VariantControl=Variant
  CANTransmit4 : ec5744lib/RapidECU_U3/04CANCommunication/CANTransmit  canmodule=0  canbuffer=8  canmessageid=hex2dec('8B1EF21')  canmessagetype=Standard(11-bit ID)  datalength=8  sampletime=-1
      settings: SourceProductName=ECUCoder for MPC5744
  MeaModule : ec5744lib/RapidECU_U3/07Calibration/MeaModule  signal=VCUtoMCU2
      settings: SourceProductName=ECUCoder for MPC5744
  Terminator3 : Terminator
  wires:
  CANTransmit4/1 -> MeaModule/1
  MeaModule/1 -> Terminator3/1
  In1/1 -> CANTransmit4/1

== system version5/output/VCUtoMCU/Subsystem1 ==
  In1 : Inport
  function : TriggerPort  TriggerType=function-call  VariantControl=Variant
  CANTransmit3 : ec5744lib/RapidECU_U3/04CANCommunication/CANTransmit  canmodule=0  canbuffer=8  canmessageid=hex2dec('8C1EF21')  canmessagetype=Standard(11-bit ID)  datalength=8  sampletime=-1
      settings: SourceProductName=ECUCoder for MPC5744
  MeaModule1 : ec5744lib/RapidECU_U3/07Calibration/MeaModule  signal=VCUtoMCU1
      settings: SourceProductName=ECUCoder for MPC5744
  Terminator2 : Terminator
  wires:
  CANTransmit3/1 -> MeaModule1/1
  MeaModule1/1 -> Terminator2/1
  In1/1 -> CANTransmit3/1

== system version5/control/APS_Ctrl/clock/计时计数 ==
  计数状态 : Inport
  Delay : Delay  DelayLength=1
  MATLAB Function : MATLAB Function  TreatAsAtomicUnit=on
  计数次数 : Constant  Value=5  SampleTime=-1
  Count_state : Outport
  wires:
  MATLAB Function/2(y) -> Delay/1
  Delay/1 -> MATLAB Function/3(old_u)
  MATLAB Function/1(Bukekao) -> Count_state/1
  计数状态/1 -> MATLAB Function/1(u)
  计数次数/1 -> MATLAB Function/2(continuous_num)

== system version5/input/BMStoVCU/Function-Call Subsystem/Enabled Subsystem ==
  ID : Inport
  Msg : Inport  Port=2
  Enable : EnablePort
  CAN Unpack : canmsglib/CAN Unpack  CANdbFile=C:\WH\MC.dbc  MsgList=BMStoVCU_batstat  MsgName=BMStoVCU_batstat  MsgIDType=Extended (29-bit identifier)  MsgIdentifier=408961267  MsgLength=8  SignalInfo=Bat_Ala_Lv$44$4$1$2$1$0$1$0$0$15$#Bat_Current_LSB$24$8$1$2$1$0$1.000000e-01$-1000$-1000$-9.745000e+02$#Bat_Current_MSB$16$8$1$2$1$0$1.000000e-01$-1000$-1000$-9.745000e+02$#Bat_Stat$52$4$1$2$1$0$1$0$0$15$#Bat_Voltage_LSB$8$8$1$2$1$0$1.000000e-01$0$0$2.550000e+01$#Bat_Voltage_MSB$0$8$1$2$1$0$1.000000e-01$0$0$2.550000e+01$#Bat_soc$32$8$1$2$1$0$1$0$0$255$#  NSignals=7  IDPort=off  TimestampPort=off  ErrorPort=off  RemotePort=off  LengthPort=off  StatusPort=off  StartBits=str2num('[int32(44);int32(24);int32(16);int32(52);int32(8);int32(0);int32(32)]')  SignalSizes=str2num('[int32(4);int32(8);int32(8);int32(4);int32(8);int32(8);int32(8)]')  ByteOrders=str2num('[int32(1);int32(1);int32(1);int32(1);int32(1);int32(1);int32(1)]')  DataTypes=str2num('[int32(2);int32(2);int32(2);int32(2);int32(2);int32(2);int32(2)]')  MultiplexTypes=str2num('[int32(1);int32(1);int32(1);int32(1);int32(1);int32(1);int32(1)]')  MultiplexValues=str2num('[double(0);double(0);double(0);double(0);double(0);double(0);double(0)]')  Factors=str2num('[double(1);double(1.000000e-01);double(1.000000e-01);double(1);double(1.000000e-01);double(1.000000e-01);double(1)]')  Offsets=str2num('[double(0);double(-1000);double(-1000);double(0);double(0);double(0);double(0)]')  Minimums=str2num('[double(0);double(-1000);double(-1000);double(0);double(0);double(0);double(0)]')  Maximums=str2num('[double(15);double(-9.745000e+02);double(-9.745000e+02);double(15);double(2.550000e+01);double(2.550000e+01);double(255)]')  ApplyMinMax=off
      settings: SourceProductName=Simulink Real-Time  SourceProductBaseCode=XP  DataFormat=CANdb specified signals
  CANUnPackMessage1 : ec5744lib/RapidECU_U3/04CANCommunication/CANUnPackMessage  datalength=8  canmessagetype=Extended(29-bit ID)  sampletime=-1
      settings: SourceProductName=ECUCoder for MPC5744
  Bat_Ala_Lv : Outport
  Bat_Current_LSB : Outport  Port=2
  Bat_Current_MSB : Outport  Port=3
  Bat_Stat : Outport  Port=4
  Bat_Voltage_LSB : Outport  Port=5
  Bat_Valtage_MSB : Outport  Port=6
  Bat_soc : Outport  Port=7
  wires:
  CAN Unpack/7 -> Bat_soc/1
  Msg/1 -> CANUnPackMessage1/2
  CANUnPackMessage1/1 -> CAN Unpack/1
  CAN Unpack/5 -> Bat_Voltage_LSB/1
  ID/1 -> CANUnPackMessage1/1
  CAN Unpack/3 -> Bat_Current_MSB/1
  CAN Unpack/4 -> Bat_Stat/1
  CAN Unpack/1 -> Bat_Ala_Lv/1
  CAN Unpack/6 -> Bat_Valtage_MSB/1
  CAN Unpack/2 -> Bat_Current_LSB/1

== system version5/input/BMStoVCU/Function-Call Subsystem1/Enabled Subsystem ==
  ID : Inport
  Msg : Inport  Port=2
  Enable : EnablePort
  CAN Unpack : canmsglib/CAN Unpack  CANdbFile=C:\WH\MC.dbc  MsgList=BMStoVCU_tempctrl  MsgName=BMStoVCU_tempctrl  MsgIDType=Extended (29-bit identifier)  MsgIdentifier=409092339  MsgLength=8  SignalInfo=Bat_Cooling_Ctrl$32$8$1$2$1$0$1$0$0$255$#Bat_Cooling_Ctrl_NO$16$8$1$2$1$0$1$0$0$255$#Bat_Heating_Ctrl$40$8$1$2$1$0$1$0$0$255$#Bat_Heating_Ctrl_NO$24$8$1$2$1$0$1$0$0$255$#Bat_Max_Temp$0$8$1$2$1$0$1$-40$-40$215$#Bat_Mix_Temp$8$8$1$2$1$0$1$-40$-40$215$#  NSignals=6  IDPort=off  TimestampPort=off  ErrorPort=off  RemotePort=off  LengthPort=off  StatusPort=off  StartBits=str2num('[int32(32);int32(16);int32(40);int32(24);int32(0);int32(8)]')  SignalSizes=str2num('[int32(8);int32(8);int32(8);int32(8);int32(8);int32(8)]')  ByteOrders=str2num('[int32(1);int32(1);int32(1);int32(1);int32(1);int32(1)]')  DataTypes=str2num('[int32(2);int32(2);int32(2);int32(2);int32(2);int32(2)]')  MultiplexTypes=str2num('[int32(1);int32(1);int32(1);int32(1);int32(1);int32(1)]')  MultiplexValues=str2num('[double(0);double(0);double(0);double(0);double(0);double(0)]')  Factors=str2num('[double(1);double(1);double(1);double(1);double(1);double(1)]')  Offsets=str2num('[double(0);double(0);double(0);double(0);double(-40);double(-40)]')  Minimums=str2num('[double(0);double(0);double(0);double(0);double(-40);double(-40)]')  Maximums=str2num('[double(255);double(255);double(255);double(255);double(215);double(215)]')  ApplyMinMax=off
      settings: SourceProductName=Simulink Real-Time  SourceProductBaseCode=XP  DataFormat=CANdb specified signals
  CANUnPackMessage : ec5744lib/RapidECU_U3/04CANCommunication/CANUnPackMessage  datalength=8  canmessagetype=Standard(11-bit ID)  sampletime=-1
      settings: SourceProductName=ECUCoder for MPC5744
  Terminator{,1..4} (5 alike) : Terminator
  Bat_Max_Temp : Outport
  wires:
  Msg/1 -> CANUnPackMessage/2
  CANUnPackMessage/1 -> CAN Unpack/1
  ID/1 -> CANUnPackMessage/1
  CAN Unpack/5 -> Bat_Max_Temp/1
  CAN Unpack/1 -> Terminator4/1
  CAN Unpack/2 -> Terminator3/1
  CAN Unpack/3 -> Terminator2/1
  CAN Unpack/4 -> Terminator1/1
  CAN Unpack/6 -> Terminator/1

== system version5/input/DASHtoVCU/Function-Call Subsystem6/Enabled Subsystem ==
  ID : Inport
  Msg : Inport  Port=2
  Enable : EnablePort
  CAN Unpack : canmsglib/CAN Unpack  CANdbFile=C:\WH\MC.dbc  MsgList=DashtoVCU  MsgName=DashtoVCU  MsgIDType=Standard (11-bit identifier)  MsgIdentifier=528  MsgLength=8  SignalInfo=GEAR$0$2$1$2$1$0$1$0$0$3$#Key_For_Dash$8$8$1$2$1$0$1$0$0$255$#  NSignals=2  IDPort=off  TimestampPort=off  ErrorPort=off  RemotePort=off  LengthPort=off  StatusPort=off  StartBits=str2num('[int32(0);int32(8)]')  SignalSizes=str2num('[int32(2);int32(8)]')  ByteOrders=str2num('[int32(1);int32(1)]')  DataTypes=str2num('[int32(2);int32(2)]')  MultiplexTypes=str2num('[int32(1);int32(1)]')  MultiplexValues=str2num('[double(0);double(0)]')  Factors=str2num('[double(1);double(1)]')  Offsets=str2num('[double(0);double(0)]')  Minimums=str2num('[double(0);double(0)]')  Maximums=str2num('[double(3);double(255)]')  ApplyMinMax=off
      settings: SourceProductName=Simulink Real-Time  SourceProductBaseCode=XP  DataFormat=CANdb specified signals
  CANUnPackMessage : ec5744lib/RapidECU_U3/04CANCommunication/CANUnPackMessage  datalength=8  canmessagetype=Standard(11-bit ID)  sampletime=-1
      settings: SourceProductName=ECUCoder for MPC5744
  GEAR : Outport
  Key_For_Dash : Outport  Port=2
  wires:
  ID/1 -> CANUnPackMessage/1
  CANUnPackMessage/1 -> CAN Unpack/1
  Msg/1 -> CANUnPackMessage/2
  CAN Unpack/1 -> GEAR/1
  CAN Unpack/2 -> Key_For_Dash/1

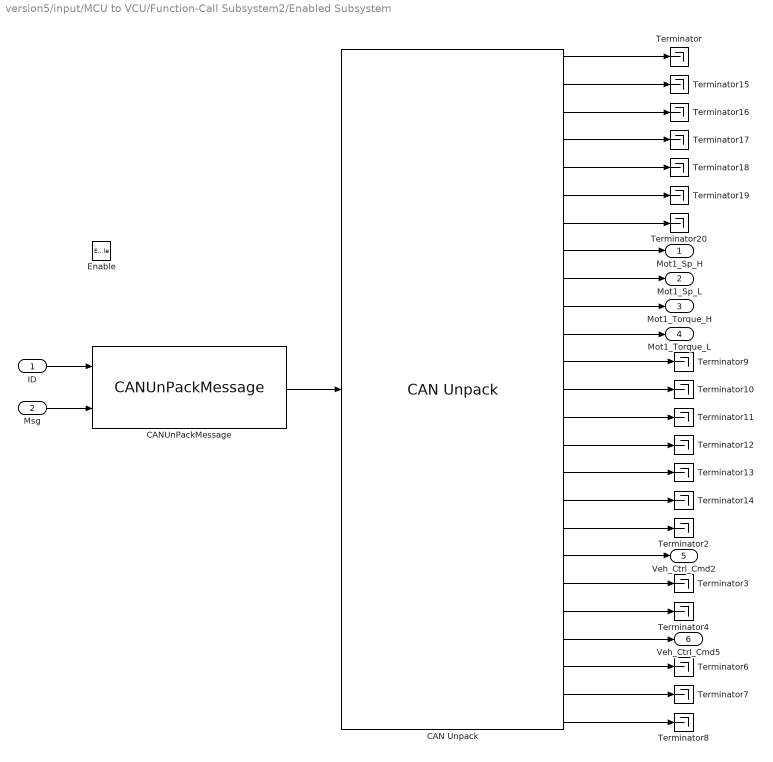
== system version5/input/MCU to VCU/Function-Call Subsystem2/Enabled Subsystem ==
  ID : Inport
  Msg : Inport  Port=2
  Enable : EnablePort
  CAN Unpack : canmsglib/CAN Unpack  CANdbFile=C:\WH\MC.dbc  MsgList=MCU1toVCU1_Ctrl  MsgName=MCU1toVCU1_Ctrl  MsgIDType=Extended (29-bit identifier)  MsgIdentifier=218089199  MsgLength=8  SignalInfo=Alarm_Reserved_Bit$50$1$1$2$1$0$1$0$0$1$#Bus_Over_Voltage$44$1$1$2$1$0$1$0$0$1$#Bus_Under_Voltage$46$1$1$2$1$0$1$0$0$1$#Combined_Alarm$56$2$1$2$1$0$1$0$0$3$#Control_Circuit_Anomaly$45$1$1$2$1$0$1$0$0$1$#Controller_Temp_Ala$48$1$1$2$1$0$1$0$0$1$#Ctrl_Rd$40$1$1$2$1$0$1$0$0$1$#Mot1_Sp_H$16$8$1$2$1$0$5.000000e-01$-10000$-10000$-9.872500e+03$#Mot1_Sp_L$24$8$1$2$1$0$5.000000e-01$-10000$-10064$-9.936500e+03$#Mot1_Torque_H$0$8$1$2$1$0$5.000000e-01$-10000$-10000$-9.872500e+03$#Mot1_Torque_L$8$8$1$2$1$0$5.000000e-01$-10000$-10000$-9.872500e+03$#Motor_Temp_Ala$49$1$1$2$1$0$1$0$0$1$#Over_Current$43$1$1$2$1$0$1$0$0$1$#Power_Limit$47$1$1$2$1$0$1$0$0$1$#Precharge_Condition$41$1$1$2$1$0$1$0$0$1$#Rotatory_Sen$42$1$1$2$1$0$1$0$0$1$#Self_Check$55$1$1$2$1$0$1$0$0$1$#Veh_Ctrl_Cmd1$32$1$1$2$1$0$1$0$0$1$#Veh_Ctrl_Cmd2$33$1$1$2$1$0$1$0$0$1$#Veh_Ctrl_Cmd3$34$1$1$2$1$0$1$0$0$1$#Veh_Ctrl_Cmd4$35$1$1$2$1$0$1$0$0$1$#Veh_Ctrl_Cmd5$36$1$1$2$1$0$1$0$0$1$#Veh_Ctrl_Cmd6$37$1$1$2$1$0$1$0$0$1$#Veh_Ctrl_Cmd7$38$1$1$2$1$0$1$0$0$1$#Veh_Ctrl_Cmd8$39$1$1$2$1$0$1$0$0$1$#  NSignals=25  IDPort=off  TimestampPort=off  ErrorPort=off  RemotePort=off  LengthPort=off  StatusPort=off  StartBits=str2num('[int32(50);int32(44);int32(46);int32(56);int32(45);int32(48);int32(40);int32(16);int32(24);int32(0);int32(8);int32(49);int32(43);int32(47);int32(41);int32(42);int32(55);int32(32);int32(33);int32(34);int32(35);int32(36);int32(37);int32(38);int32(39)]')  SignalSizes=str2num('[int32(1);int32(1);int32(1);int32(2);int32(1);int32(1);int32(1);int32(8);int32(8);int32(8);int32(8);int32(1);int32(1);int32(1);int32(1);int32(1);int32(1);int32(1);int32(1);int32(1);int32(1);int32(1);int32(1);int32(1);int32(1)]')  ByteOrders=str2num('[int32(1);int32(1);int32(1);int32(1);int32(1);int32(1);int32(1);int32(1);int32(1);int32(1);int32(1);int32(1);int32(1);int32(1);int32(1);int32(1);int32(1);int32(1);int32(1);int32(1);int32(1);int32(1);int32(1);int32(1);int32(1)]')  DataTypes=str2num('[int32(2);int32(2);int32(2);int32(2);int32(2);int32(2);int32(2);int32(2);int32(2);int32(2);int32(2);int32(2);int32(2);int32(2);int32(2);int32(2);int32(2);int32(2);int32(2);int32(2);int32(2);int32(2);int32(2);int32(2);int32(2)]')  MultiplexTypes=str2num('[int32(1);int32(1);int32(1);int32(1);int32(1);int32(1);int32(1);int32(1);int32(1);int32(1);int32(1);int32(1);int32(1);int32(1);int32(1);int32(1);int32(1);int32(1);int32(1);int32(1);int32(1);int32(1);int32(1);int32(1);int32(1)]')  MultiplexValues=str2num('[double(0);double(0);double(0);double(0);double(0);double(0);double(0);double(0);double(0);double(0);double(0);double(0);double(0);double(0);double(0);double(0);double(0);double(0);double(0);double(0);double(0);double(0);double(0);double(0);double(0)]')  Factors=str2num('[double(1);double(1);double(1);double(1);double(1);double(1);double(1);double(5.000000e-01);double(5.000000e-01);double(5.000000e-01);double(5.000000e-01);double(1);double(1);double(1);double(1);double(1);double(1);double(1);double(1);double(1);double(1);double(1);double(1);double(1);double(1)]')  Offsets=str2num('[double(0);double(0);double(0);double(0);double(0);double(0);double(0);double(-10000);double(-10000);double(-10000);double(-10000);double(0);double(0);double(0);double(0);double(0);double(0);double(0);double(0);double(0);double(0);double(0);double(0);double(0);double(0)]')  Minimums=str2num('[double(0);double(0);double(0);double(0);double(0);double(0);double(0);double(-10000);double(-10064);double(-10000);double(-10000);double(0);double(0);double(0);double(0);double(0);double(0);double(0);double(0);double(0);double(0);double(0);double(0);double(0);double(0)]')  Maximums=str2num('[double(1);double(1);double(1);double(3);double(1);double(1);double(1);double(-9.872500e+03);double(-9.936500e+03);double(-9.872500e+03);double(-9.872500e+03);double(1);double(1);double(1);double(1);double(1);double(1);double(1);double(1);double(1);double(1);double(1);double(1);double(1);double(1)]')  ApplyMinMax=off
      settings: SourceProductName=Simulink Real-Time  SourceProductBaseCode=XP  DataFormat=CANdb specified signals
  CANUnPackMessage : ec5744lib/RapidECU_U3/04CANCommunication/CANUnPackMessage  datalength=8  canmessagetype=Standard(11-bit ID)  sampletime=-1
      settings: SourceProductName=ECUCoder for MPC5744
  Terminator{,2..4,6..20} (19 alike) : Terminator
  Mot1_Sp_H : Outport
  Mot1_Sp_L : Outport  Port=2
  Mot1_Torque_H : Outport  Port=3
  Mot1_Torque_L : Outport  Port=4
  Veh_Ctrl_Cmd2 : Outport  Port=5
  Veh_Ctrl_Cmd5 : Outport  Port=6
  wires:
  Msg/1 -> CANUnPackMessage/2
  CANUnPackMessage/1 -> CAN Unpack/1
  ID/1 -> CANUnPackMessage/1
  CAN Unpack/8 -> Mot1_Sp_H/1
  CAN Unpack/9 -> Mot1_Sp_L/1
  CAN Unpack/11 -> Mot1_Torque_L/1
  CAN Unpack/10 -> Mot1_Torque_H/1
  CAN Unpack/18 -> Terminator2/1
  CAN Unpack/19 -> Veh_Ctrl_Cmd2/1
  CAN Unpack/20 -> Terminator3/1
  CAN Unpack/21 -> Terminator4/1
  CAN Unpack/22 -> Veh_Ctrl_Cmd5/1
  CAN Unpack/23 -> Terminator6/1
  CAN Unpack/24 -> Terminator7/1
  CAN Unpack/25 -> Terminator8/1
  CAN Unpack/12 -> Terminator9/1
  CAN Unpack/13 -> Terminator10/1
  CAN Unpack/14 -> Terminator11/1
  CAN Unpack/15 -> Terminator12/1
  CAN Unpack/16 -> Terminator13/1
  CAN Unpack/17 -> Terminator14/1
  CAN Unpack/4 -> Terminator17/1
  CAN Unpack/3 -> Terminator16/1
  CAN Unpack/2 -> Terminator15/1
  CAN Unpack/1 -> Terminator/1
  CAN Unpack/5 -> Terminator18/1
  CAN Unpack/6 -> Terminator19/1
  CAN Unpack/7 -> Terminator20/1
